simulink model "gocontroll_demo"  (R2025a)
settings: Solver=FixedStepDiscrete  StartTime=0.0  StopTime=5  FixedStep=0.01  RelTol=1e-3
PostLoadFcn:
  | try
  |     eval([bdroot,'_startup']) %to run model_startup.m
  | catch
  |     disp("No startup file found for this model");
  | end
  | core_info = evalc('feature(''numcores'')');
  | core_info_split = split(core_info, " ");
  | num_cores = core_info_split{12};
  | set_param(bdroot, "MakeCommand", ['make_rtw -j' num_cores]);
  | clear num_cores core_info core_info_split
values from neighbouring files (symbols this model uses):
  DisplayBrightness = Simulink.Parameter    [gocontroll_demo_startup.m]
libraries: GOcontroll_Moduline_Target x4
settings Model: Creator=maud  LastModifiedBy=maud
settings SolverCC: AlgebraicLoopSolver=TrustRegion
settings DataIOCC: LimitDataPoints=on  SaveFormat=Array  ReturnWorkspaceOutputs=off
settings OptimizationCC: BlockReduction=off  DefaultParameterBehavior=Inlined  EnhancedBackFolding=on  CachingGlobalReferences=on  LifeSpan=1  OptimizeBlockOrder=speed  EfficientTunableParamExpr=on
settings DebuggingCC: SolverPrmCheckMsg=warning  InheritedTsInSrcMsg=none  MultiTaskRateTransMsg=warning  ParameterPrecisionLossMsg=none  UnconnectedInputMsg=error  UnconnectedOutputMsg=error  UnconnectedLineMsg=error  SFUnusedDataAndEventsDiag=none  SFUnexpectedBacktrackingDiag=warning  SFNoUnconditionalDefaultTransitionDiag=warning  SFUndirectedBroadcastEventsDiag=none  SFExecutionAtInitializationDiag=none  RCSCRenamedMsg=none  RCSCObservableMsg=none  ArithmeticOperatorsInVariantConditions=warning
settings HardwareCC: ProdBitPerLong=64.0  ProdLargestAtomicInteger=LongLong  ProdLargestAtomicFloat=Double  ProdLongLongMode=on  ProdHWDeviceType=ARM Compatible->ARM 64-bit (LP64)
settings ModelReferenceCC: EnableRefExpFcnMdlSchedulingChecks=on  PropagateSignalLabelsOutOfModel=off
settings SFSimCC: SimUseLocalCustomCode=off  MATLABDynamicMemAlloc=off  CustomCodeUndefinedFunction=UseInterfaceOnly
settings RTWCC: SystemTargetFile=ert_linux.tlc  MakeCommand=make_rtw -j24  TemplateMakefile=ert_linux_target_64.tmf  RetainRTWFile=on  RTWUseLocalCustomCode=off  GPUComputeCapability=3.5  Description=Linux Embedded Coder
settings CodeAppCC: IgnoreCustomStorageClasses=off  StateflowObjectComments=on
settings STFCustomTargetCC: SystemTargetFile=ert_linux.tlc  CodeReplacementLibrary=GNU C99 extensions  MultiwordLength=2048.0  DynamicStringBufferSize=256.0  CombineOutputUpdateFcns=on  ERTCustomFileBanners=on  SupportContinuousTime=off  SupportNonInlinedSFcns=off  RemoveResetFunc=on  MATLABClassNameForMDSCustomization=Simulink.SoftwareTarget.ERTCustomization  GRTInterface=off  tlcAutoUpload=Do not upload  tlcLinuxPriority=40.0  tlcLinuxTarget=i.MX8  tlcXcpTcpAddress=192.168.19.85  tlcUploadPort=8001.0  tlcLinuxCompiler=GCC  tlcXcpTcpPort=50002.0
settings ERTTargetCC: ExtModeTransport=0.0  ExtModeStaticAlloc=off  ExtModeMexFile=ext_comm  ExtModeIntrfLevel=Level1  InlinedParameterPlacement=Hierarchical  ERTCustomFileTemplate=ert_linux_file_process.tlc  PreserveExpressionOrder=on  SuppressUnreachableDefaultCases=off  DynamicArrayContainerType=coder::array  CodeReplacementLibrary=GNU C99 extensions  MultiwordLength=2048.0  ParMdlRefBuildCompliant=off  CompOptLevelCompliant=off  ConcurrentExecutionCompliant=off  ModelStepFunctionPrototypeControlCompliant=off  CPPClassGenCompliant=off  UseToolchainInfoCompliant=off
settings ConfigComp: CovMetricSettings=dw  CovSaveCumulativeToWorkspaceVar=on  CovSaveSingleToWorkspaceVar=on  CovExternalEMLEnable=off  CovSFcnEnable=off
settings SimscapeCC: SimscapeLogDataHistory=5000  SimscapeLogDecimation=1

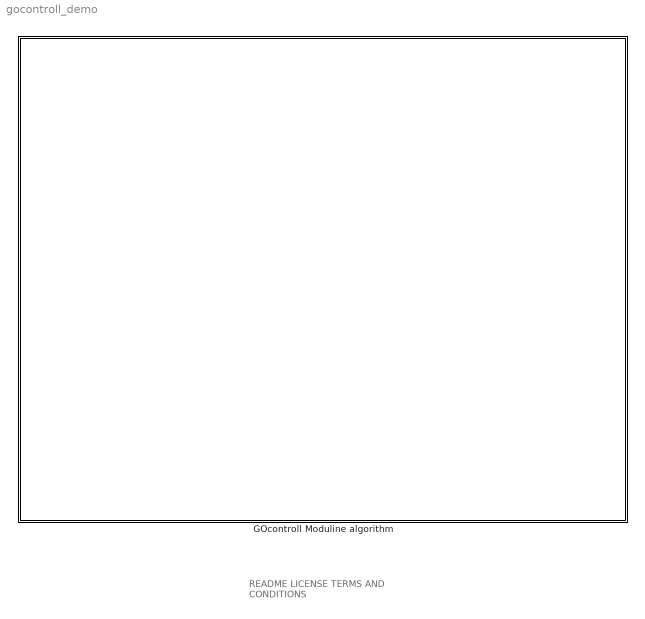
== system gocontroll_demo ==
  note: README
      |
      | LICENSE
      |
      | TERMS AND CONDITIONS
  GOcontroll Moduline algorithm : Subsystem  mask(TopLevelSubsystem){}
      mask Display: image(gocontroll_png())

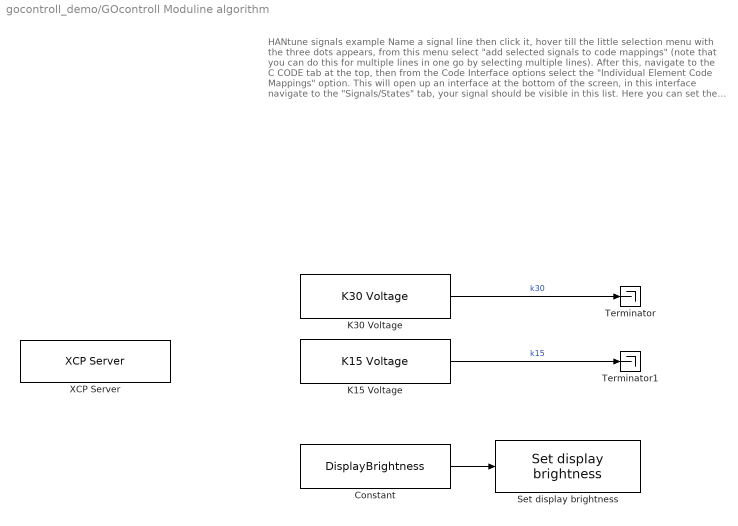
== system gocontroll_demo/GOcontroll Moduline algorithm ==
  note: HANtune signals example
      | Name a signal line then click it, hover till the little selection menu with
      | the three dots appears, from this menu select "add selected signals
      | to code mappings" (note that you can do this for multiple lines in one go
      | by selecting multiple lines).
      | After this, navigate to the C CODE tab at the top, then from the Code
      | Interface options select the "Individual Element Code Mappings" option.
      | This will open up an interface at the bottom of the screen, in this interface
      | navigate to the "Signals/States" tab, your signal should be visible in this list.
      | Here you can set the storage class to "ExportedGlobal", this can also be
      | done for multiple signals in one go by selecting multiple signals in the list
      | with ctrl or shift click, and then changing the storage class for any of the
      | selected signals.
  Constant : Constant  Value=DisplayBrightness
  K15 Voltage : GOcontroll_Moduline_Target/Supply control/K15 Voltage  Tag=HANcoder_GOcontroll_Moduline_IV  ContrType=GOcontroll Moduline Display  tsamp=0.05  k15pin=K15 (Connector A pin 9)
      settings: SourceProductName=GOcontroll Moduline
  K30 Voltage : GOcontroll_Moduline_Target/Supply control/K30 Voltage  Tag=HANcoder_GOcontroll_Moduline_IV  ContrType=GOcontroll Moduline Display  tsamp=0.05
      settings: SourceProductName=GOcontroll Moduline
  Set display brightness : GOcontroll_Moduline_Target/Display specific/Set display brightness  tsamp=1
      settings: SourceProductName=GOcontroll Moduline
  Terminator : Terminator
  Terminator1 : Terminator
  XCP Server : GOcontroll_Moduline_Target/System/XCP Server  Priority=999999  server_type=TCP
      settings: SourceProductName=GOcontroll Moduline
  wires:
  K15 Voltage/1 -> Terminator1/1  "k15"
  K30 Voltage/1 -> Terminator/1  "k30"
  Constant/1 -> Set display brightness/1
